simulink model "reference_block"  (R2016a)
settings: Solver=VariableStepAuto  StartTime=0.0  StopTime=10.0  RelTol=1e-3
libraries: robotlib x42
settings Model: Creator=rasrack  LastModifiedBy=rasrack

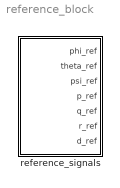
== system reference_block ==
  reference_signals : Subsystem

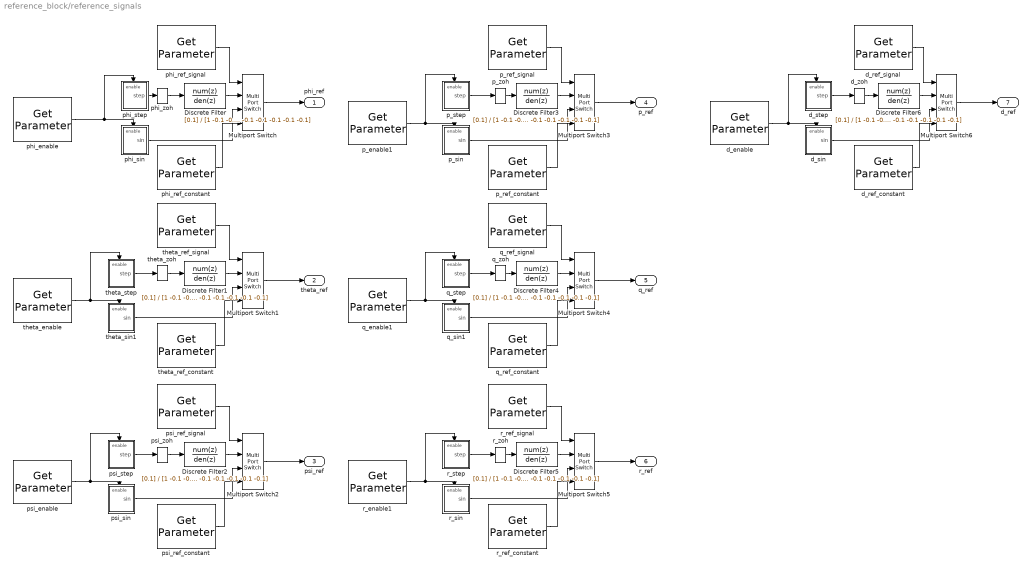
== system reference_block/reference_signals ==
  Discrete Filter{,1..6} (7 alike) : DiscreteFilter  Numerator=[0.1]  Denominator=[1 -0.1 -0.1 -0.1 -0.1 -0.1 -0.1 -0.1 -0.1 -0.1]
  Multiport Switch{,1..6} (7 alike) : MultiPortSwitch
  d_enable : robotlib/Get Parameter  SourceLibraryInfo=This block requires Robotics System Toolbox  ParameterSource=Specify your own  ParameterName=/matlab_controller/d_reference/enable  ParameterType=double  ParameterMaxArrayLength=16  ParameterInitialValue=0.0  SampleTime=-1  ShowErrorCodeOutput=off  ModelName=reference_block  BlockId=ParamGet_reference_block_242
  d_ref_constant : robotlib/Get Parameter  SourceLibraryInfo=This block requires Robotics System Toolbox  ParameterSource=Specify your own  ParameterName=/matlab_controller/d_ref_constant  ParameterType=double  ParameterMaxArrayLength=16  ParameterInitialValue=0.0  SampleTime=-1  ShowErrorCodeOutput=off  ModelName=reference_block  BlockId=ParamGet_reference_block_269
  d_ref_signal : robotlib/Get Parameter  SourceLibraryInfo=This block requires Robotics System Toolbox  ParameterSource=Specify your own  ParameterName=/matlab_controller/d_reference_signal  ParameterType=double  ParameterMaxArrayLength=16  ParameterInitialValue=0.0  SampleTime=-1  ShowErrorCodeOutput=off  ModelName=reference_block  BlockId=ParamGet_reference_block_256
  d_sin : Subsystem
  d_step : Subsystem
  d_zoh : ZeroOrderHold  SampleTime=0.010000
  p_enable1 : robotlib/Get Parameter  SourceLibraryInfo=This block requires Robotics System Toolbox  ParameterSource=Specify your own  ParameterName=/matlab_controller/p_reference/enable  ParameterType=double  ParameterMaxArrayLength=16  ParameterInitialValue=0.0  SampleTime=-1  ShowErrorCodeOutput=off  ModelName=reference_block  BlockId=ParamGet_reference_block_216
  p_ref_constant : robotlib/Get Parameter  SourceLibraryInfo=This block requires Robotics System Toolbox  ParameterSource=Specify your own  ParameterName=/matlab_controller/p_ref_constant  ParameterType=double  ParameterMaxArrayLength=16  ParameterInitialValue=0.0  SampleTime=-1  ShowErrorCodeOutput=off  ModelName=reference_block  BlockId=ParamGet_reference_block_268
  p_ref_signal : robotlib/Get Parameter  SourceLibraryInfo=This block requires Robotics System Toolbox  ParameterSource=Specify your own  ParameterName=/matlab_controller/p_reference_signal  ParameterType=double  ParameterMaxArrayLength=16  ParameterInitialValue=0.0  SampleTime=-1  ShowErrorCodeOutput=off  ModelName=reference_block  BlockId=ParamGet_reference_block_257
  p_sin : Subsystem
  p_step : Subsystem
  p_zoh : ZeroOrderHold  SampleTime=0.010000
  phi_enable : robotlib/Get Parameter  SourceLibraryInfo=This block requires Robotics System Toolbox  ParameterSource=Specify your own  ParameterName=/matlab_controller/phi_reference/enable  ParameterType=double  ParameterMaxArrayLength=16  ParameterInitialValue=0.0  SampleTime=-1  ShowErrorCodeOutput=off  ModelName=reference_block  BlockId=ParamGet_reference_block_142
  phi_ref_constant : robotlib/Get Parameter  SourceLibraryInfo=This block requires Robotics System Toolbox  ParameterSource=Specify your own  ParameterName=/matlab_controller/phi_ref_constant  ParameterType=double  ParameterMaxArrayLength=16  ParameterInitialValue=0.0  SampleTime=-1  ShowErrorCodeOutput=off  ModelName=reference_block  BlockId=ParamGet_reference_block_262
  phi_ref_signal : robotlib/Get Parameter  SourceLibraryInfo=This block requires Robotics System Toolbox  ParameterSource=Specify your own  ParameterName=/matlab_controller/phi_reference_signal  ParameterType=double  ParameterMaxArrayLength=16  ParameterInitialValue=0.0  SampleTime=-1  ShowErrorCodeOutput=off  ModelName=reference_block  BlockId=ParamGet_reference_block_255
  phi_sin : Subsystem
  phi_step : Subsystem
  phi_zoh : ZeroOrderHold  SampleTime=0.010000
  psi_enable : robotlib/Get Parameter  SourceLibraryInfo=This block requires Robotics System Toolbox  ParameterSource=Specify your own  ParameterName=/matlab_controller/psi_reference/enable  ParameterType=double  ParameterMaxArrayLength=16  ParameterInitialValue=0.0  SampleTime=-1  ShowErrorCodeOutput=off  ModelName=reference_block  BlockId=ParamGet_reference_block_164
  psi_ref_constant : robotlib/Get Parameter  SourceLibraryInfo=This block requires Robotics System Toolbox  ParameterSource=Specify your own  ParameterName=/matlab_controller/psi_ref_constant  ParameterType=double  ParameterMaxArrayLength=16  ParameterInitialValue=0.0  SampleTime=-1  ShowErrorCodeOutput=off  ModelName=reference_block  BlockId=ParamGet_reference_block_265
  psi_ref_signal : robotlib/Get Parameter  SourceLibraryInfo=This block requires Robotics System Toolbox  ParameterSource=Specify your own  ParameterName=/matlab_controller/psi_reference_signal  ParameterType=double  ParameterMaxArrayLength=16  ParameterInitialValue=0.0  SampleTime=-1  ShowErrorCodeOutput=off  ModelName=reference_block  BlockId=ParamGet_reference_block_260
  psi_sin : Subsystem
  psi_step : Subsystem
  psi_zoh : ZeroOrderHold  SampleTime=0.010000
  q_enable1 : robotlib/Get Parameter  SourceLibraryInfo=This block requires Robotics System Toolbox  ParameterSource=Specify your own  ParameterName=/matlab_controller/q_reference/enable  ParameterType=double  ParameterMaxArrayLength=16  ParameterInitialValue=0.0  SampleTime=-1  ShowErrorCodeOutput=off  ModelName=reference_block  BlockId=ParamGet_reference_block_203
  q_ref_constant : robotlib/Get Parameter  SourceLibraryInfo=This block requires Robotics System Toolbox  ParameterSource=Specify your own  ParameterName=/matlab_controller/q_ref_constant  ParameterType=double  ParameterMaxArrayLength=16  ParameterInitialValue=0.0  SampleTime=-1  ShowErrorCodeOutput=off  ModelName=reference_block  BlockId=ParamGet_reference_block_267
  q_ref_signal : robotlib/Get Parameter  SourceLibraryInfo=This block requires Robotics System Toolbox  ParameterSource=Specify your own  ParameterName=/matlab_controller/q_reference_signal  ParameterType=double  ParameterMaxArrayLength=16  ParameterInitialValue=0.0  SampleTime=-1  ShowErrorCodeOutput=off  ModelName=reference_block  BlockId=ParamGet_reference_block_258
  q_sin1 : Subsystem
  q_step : Subsystem
  q_zoh : ZeroOrderHold  SampleTime=0.010000
  r_enable1 : robotlib/Get Parameter  SourceLibraryInfo=This block requires Robotics System Toolbox  ParameterSource=Specify your own  ParameterName=/matlab_controller/r_reference/enable  ParameterType=double  ParameterMaxArrayLength=16  ParameterInitialValue=0.0  SampleTime=-1  ShowErrorCodeOutput=off  ModelName=reference_block  BlockId=ParamGet_reference_block_190
  r_ref_constant : robotlib/Get Parameter  SourceLibraryInfo=This block requires Robotics System Toolbox  ParameterSource=Specify your own  ParameterName=/matlab_controller/r_ref_constant  ParameterType=double  ParameterMaxArrayLength=16  ParameterInitialValue=0.0  SampleTime=-1  ShowErrorCodeOutput=off  ModelName=reference_block  BlockId=ParamGet_reference_block_266
  r_ref_signal : robotlib/Get Parameter  SourceLibraryInfo=This block requires Robotics System Toolbox  ParameterSource=Specify your own  ParameterName=/matlab_controller/r_reference_signal  ParameterType=double  ParameterMaxArrayLength=16  ParameterInitialValue=0.0  SampleTime=-1  ShowErrorCodeOutput=off  ModelName=reference_block  BlockId=ParamGet_reference_block_259
  r_sin : Subsystem
  r_step : Subsystem
  r_zoh : ZeroOrderHold  SampleTime=0.010000
  theta_enable : robotlib/Get Parameter  SourceLibraryInfo=This block requires Robotics System Toolbox  ParameterSource=Specify your own  ParameterName=/matlab_controller/theta_reference/enable  ParameterType=double  ParameterMaxArrayLength=16  ParameterInitialValue=0.0  SampleTime=-1  ShowErrorCodeOutput=off  ModelName=reference_block  BlockId=ParamGet_reference_block_151
  theta_ref_constant : robotlib/Get Parameter  SourceLibraryInfo=This block requires Robotics System Toolbox  ParameterSource=Specify your own  ParameterName=/matlab_controller/theta_ref_constant  ParameterType=double  ParameterMaxArrayLength=16  ParameterInitialValue=0.0  SampleTime=-1  ShowErrorCodeOutput=off  ModelName=reference_block  BlockId=ParamGet_reference_block_264
  theta_ref_signal : robotlib/Get Parameter  SourceLibraryInfo=This block requires Robotics System Toolbox  ParameterSource=Specify your own  ParameterName=/matlab_controller/theta_reference_signal  ParameterType=double  ParameterMaxArrayLength=16  ParameterInitialValue=0.0  SampleTime=-1  ShowErrorCodeOutput=off  ModelName=reference_block  BlockId=ParamGet_reference_block_261
  theta_sin1 : Subsystem
  theta_step : Subsystem
  theta_zoh : ZeroOrderHold  SampleTime=0.010000
  phi_ref : Outport
  theta_ref : Outport  Port=2
  psi_ref : Outport  Port=3
  p_ref : Outport  Port=4
  q_ref : Outport  Port=5
  r_ref : Outport  Port=6
  d_ref : Outport  Port=7
  wires:
  psi_enable/1 -> psi_step/Enable, psi_sin/Enable
  p_ref_constant/1 -> Multiport Switch3/4
  theta_ref_constant/1 -> Multiport Switch1/4
  p_sin/1(sin) -> Multiport Switch3/3
  Multiport Switch/1 -> phi_ref/1
  Discrete Filter/1 -> Multiport Switch/2
  phi_sin/1(sin) -> Multiport Switch/3
  phi_ref_signal/1 -> Multiport Switch/1
  phi_ref_constant/1 -> Multiport Switch/4
  Discrete Filter1/1 -> Multiport Switch1/2
  theta_sin1/1(sin) -> Multiport Switch1/3
  theta_ref_signal/1 -> Multiport Switch1/1
  Multiport Switch1/1 -> theta_ref/1
  Multiport Switch2/1 -> psi_ref/1
  Discrete Filter2/1 -> Multiport Switch2/2
  psi_ref_signal/1 -> Multiport Switch2/1
  Multiport Switch3/1 -> p_ref/1
  Discrete Filter3/1 -> Multiport Switch3/2
  p_ref_signal/1 -> Multiport Switch3/1
  Discrete Filter4/1 -> Multiport Switch4/2
  q_ref_signal/1 -> Multiport Switch4/1
  Multiport Switch4/1 -> q_ref/1
  Multiport Switch5/1 -> r_ref/1
  Discrete Filter5/1 -> Multiport Switch5/2
  r_ref_signal/1 -> Multiport Switch5/1
  Multiport Switch6/1 -> d_ref/1
  Discrete Filter6/1 -> Multiport Switch6/2
  d_ref_signal/1 -> Multiport Switch6/1
  phi_step/1(step) -> phi_zoh/1
  phi_zoh/1 -> Discrete Filter/1
  theta_step/1(step) -> theta_zoh/1
  theta_zoh/1 -> Discrete Filter1/1
  psi_zoh/1 -> Discrete Filter2/1
  p_zoh/1 -> Discrete Filter3/1
  q_zoh/1 -> Discrete Filter4/1
  r_zoh/1 -> Discrete Filter5/1
  d_zoh/1 -> Discrete Filter6/1
  d_sin/1(sin) -> Multiport Switch6/3
  p_enable1/1 -> p_step/Enable, p_sin/Enable
  p_step/1(step) -> p_zoh/1
  r_ref_constant/1 -> Multiport Switch5/4
  q_step/1(step) -> q_zoh/1
  phi_enable/1 -> phi_step/Enable, phi_sin/Enable
  q_ref_constant/1 -> Multiport Switch4/4
  q_sin1/1(sin) -> Multiport Switch4/3
  psi_ref_constant/1 -> Multiport Switch2/4
  d_enable/1 -> d_step/Enable, d_sin/Enable
  theta_enable/1 -> theta_step/Enable, theta_sin1/Enable
  d_step/1(step) -> d_zoh/1
  psi_sin/1(sin) -> Multiport Switch2/3
  r_enable1/1 -> r_step/Enable, r_sin/Enable
  psi_step/1(step) -> psi_zoh/1
  d_ref_constant/1 -> Multiport Switch6/4
  r_sin/1(sin) -> Multiport Switch5/3
  q_enable1/1 -> q_step/Enable, q_sin1/Enable
  r_step/1(step) -> r_zoh/1

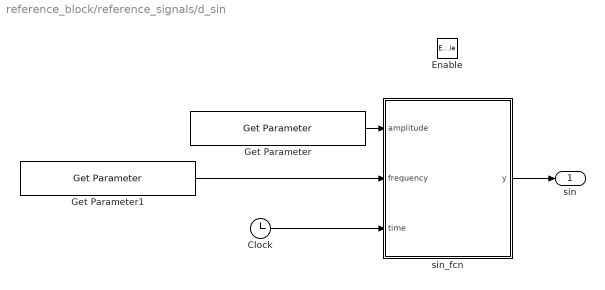
== system reference_block/reference_signals/d_sin ==
  Enable : EnablePort  StatesWhenEnabling=reset
  Clock : Clock
  Get Parameter : robotlib/Get Parameter  SourceLibraryInfo=This block requires Robotics System Toolbox  ParameterSource=Specify your own  ParameterName=/matlab_controller/d_sin/amplitude  ParameterType=double  ParameterMaxArrayLength=16  ParameterInitialValue=0.0  SampleTime=-1  ShowErrorCodeOutput=off  ModelName=reference_block  BlockId=ParamGet_reference_block_246
  Get Parameter1 : robotlib/Get Parameter  SourceLibraryInfo=This block requires Robotics System Toolbox  ParameterSource=Specify your own  ParameterName=/matlab_controller/d_sin/frequency  ParameterType=double  ParameterMaxArrayLength=16  ParameterInitialValue=0.0  SampleTime=-1  ShowErrorCodeOutput=off  ModelName=reference_block  BlockId=ParamGet_reference_block_247
  sin_fcn : MATLAB Function  TreatAsAtomicUnit=on
  sin : Outport
  wires:
  Clock/1 -> sin_fcn/3(time)
  Get Parameter1/1 -> sin_fcn/2(frequency)
  sin_fcn/1(y) -> sin/1
  Get Parameter/1 -> sin_fcn/1(amplitude)

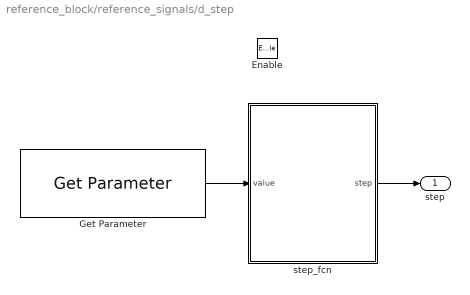
== system reference_block/reference_signals/d_step ==
  Enable : EnablePort  StatesWhenEnabling=reset
  Get Parameter : robotlib/Get Parameter  SourceLibraryInfo=This block requires Robotics System Toolbox  ParameterSource=Specify your own  ParameterName=/matlab_controller/d_step/value  ParameterType=double  ParameterMaxArrayLength=16  ParameterInitialValue=0.0  SampleTime=-1  ShowErrorCodeOutput=off  ModelName=reference_block  BlockId=ParamGet_reference_block_252
  step_fcn : MATLAB Function  TreatAsAtomicUnit=on
  step : Outport
  wires:
  step_fcn/1(step) -> step/1
  Get Parameter/1 -> step_fcn/1(value)

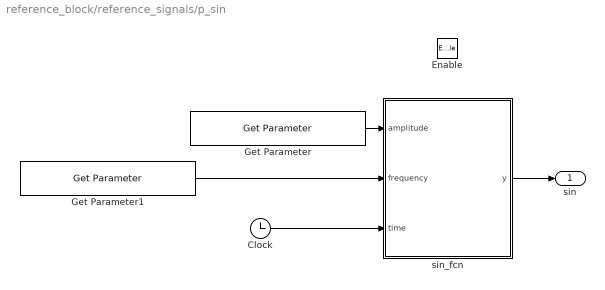
== system reference_block/reference_signals/p_sin ==
  Enable : EnablePort  StatesWhenEnabling=reset
  Clock : Clock
  Get Parameter : robotlib/Get Parameter  SourceLibraryInfo=This block requires Robotics System Toolbox  ParameterSource=Specify your own  ParameterName=/matlab_controller/p_sin/amplitude  ParameterType=double  ParameterMaxArrayLength=16  ParameterInitialValue=0.0  SampleTime=-1  ShowErrorCodeOutput=off  ModelName=reference_block  BlockId=ParamGet_reference_block_220
  Get Parameter1 : robotlib/Get Parameter  SourceLibraryInfo=This block requires Robotics System Toolbox  ParameterSource=Specify your own  ParameterName=/matlab_controller/p_sin/frequency  ParameterType=double  ParameterMaxArrayLength=16  ParameterInitialValue=0.0  SampleTime=-1  ShowErrorCodeOutput=off  ModelName=reference_block  BlockId=ParamGet_reference_block_221
  sin_fcn : MATLAB Function  TreatAsAtomicUnit=on
  sin : Outport
  wires:
  Clock/1 -> sin_fcn/3(time)
  Get Parameter1/1 -> sin_fcn/2(frequency)
  sin_fcn/1(y) -> sin/1
  Get Parameter/1 -> sin_fcn/1(amplitude)

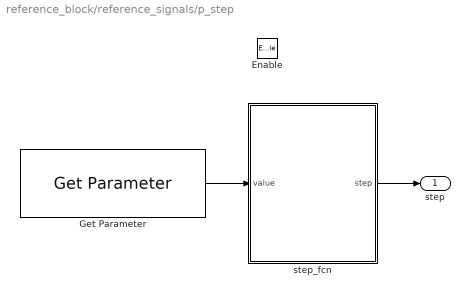
== system reference_block/reference_signals/p_step ==
  Enable : EnablePort  StatesWhenEnabling=reset
  Get Parameter : robotlib/Get Parameter  SourceLibraryInfo=This block requires Robotics System Toolbox  ParameterSource=Specify your own  ParameterName=/matlab_controller/p_step/value  ParameterType=double  ParameterMaxArrayLength=16  ParameterInitialValue=0.0  SampleTime=-1  ShowErrorCodeOutput=off  ModelName=reference_block  BlockId=ParamGet_reference_block_226
  step_fcn : MATLAB Function  TreatAsAtomicUnit=on
  step : Outport
  wires:
  step_fcn/1(step) -> step/1
  Get Parameter/1 -> step_fcn/1(value)

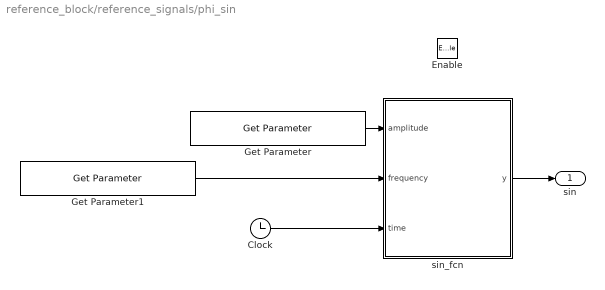
== system reference_block/reference_signals/phi_sin ==
  Enable : EnablePort  StatesWhenEnabling=reset
  Clock : Clock
  Get Parameter : robotlib/Get Parameter  SourceLibraryInfo=This block requires Robotics System Toolbox  ParameterSource=Specify your own  ParameterName=/matlab_controller/phi_sin/amplitude  ParameterType=double  ParameterMaxArrayLength=16  ParameterInitialValue=0.0  SampleTime=-1  ShowErrorCodeOutput=off  ModelName=reference_block  BlockId=ParamGet_reference_block_146
  Get Parameter1 : robotlib/Get Parameter  SourceLibraryInfo=This block requires Robotics System Toolbox  ParameterSource=Specify your own  ParameterName=/matlab_controller/phi_sin/frequency  ParameterType=double  ParameterMaxArrayLength=16  ParameterInitialValue=0.0  SampleTime=-1  ShowErrorCodeOutput=off  ModelName=reference_block  BlockId=ParamGet_reference_block_148
  sin_fcn : MATLAB Function  TreatAsAtomicUnit=on
  sin : Outport
  wires:
  Clock/1 -> sin_fcn/3(time)
  Get Parameter1/1 -> sin_fcn/2(frequency)
  sin_fcn/1(y) -> sin/1
  Get Parameter/1 -> sin_fcn/1(amplitude)

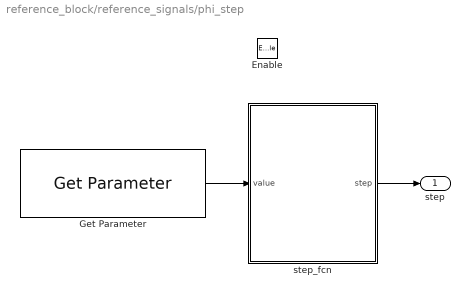
== system reference_block/reference_signals/phi_step ==
  Enable : EnablePort  StatesWhenEnabling=reset
  Get Parameter : robotlib/Get Parameter  SourceLibraryInfo=This block requires Robotics System Toolbox  ParameterSource=Specify your own  ParameterName=/matlab_controller/phi_step/value  ParameterType=double  ParameterMaxArrayLength=16  ParameterInitialValue=0.0  SampleTime=-1  ShowErrorCodeOutput=off  ModelName=reference_block  BlockId=ParamGet_reference_block_141
  step_fcn : MATLAB Function  TreatAsAtomicUnit=on
  step : Outport
  wires:
  step_fcn/1(step) -> step/1
  Get Parameter/1 -> step_fcn/1(value)

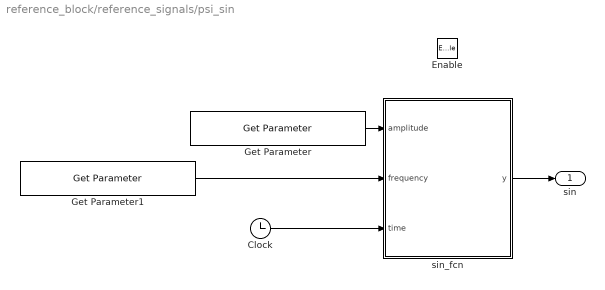
== system reference_block/reference_signals/psi_sin ==
  Enable : EnablePort  StatesWhenEnabling=reset
  Clock : Clock
  Get Parameter : robotlib/Get Parameter  SourceLibraryInfo=This block requires Robotics System Toolbox  ParameterSource=Specify your own  ParameterName=/matlab_controller/psi_sin/amplitude  ParameterType=double  ParameterMaxArrayLength=16  ParameterInitialValue=0.0  SampleTime=-1  ShowErrorCodeOutput=off  ModelName=reference_block  BlockId=ParamGet_reference_block_168
  Get Parameter1 : robotlib/Get Parameter  SourceLibraryInfo=This block requires Robotics System Toolbox  ParameterSource=Specify your own  ParameterName=/matlab_controller/psi_sin/frequency  ParameterType=double  ParameterMaxArrayLength=16  ParameterInitialValue=0.0  SampleTime=-1  ShowErrorCodeOutput=off  ModelName=reference_block  BlockId=ParamGet_reference_block_169
  sin_fcn : MATLAB Function  TreatAsAtomicUnit=on
  sin : Outport
  wires:
  Clock/1 -> sin_fcn/3(time)
  Get Parameter1/1 -> sin_fcn/2(frequency)
  sin_fcn/1(y) -> sin/1
  Get Parameter/1 -> sin_fcn/1(amplitude)

== system reference_block/reference_signals/psi_step ==
  Enable : EnablePort  StatesWhenEnabling=reset
  Get Parameter : robotlib/Get Parameter  SourceLibraryInfo=This block requires Robotics System Toolbox  ParameterSource=Specify your own  ParameterName=/matlab_controller/psi_step/value  ParameterType=double  ParameterMaxArrayLength=16  ParameterInitialValue=0.0  SampleTime=-1  ShowErrorCodeOutput=off  ModelName=reference_block  BlockId=ParamGet_reference_block_174
  step_fcn : MATLAB Function  TreatAsAtomicUnit=on
  step : Outport
  wires:
  step_fcn/1(step) -> step/1
  Get Parameter/1 -> step_fcn/1(value)

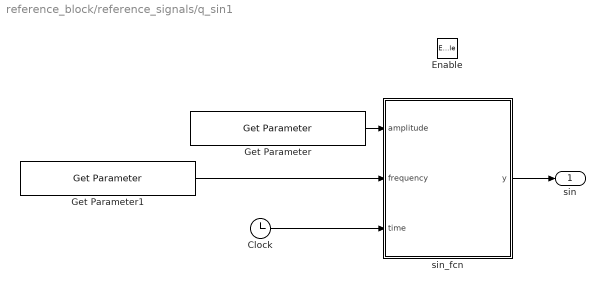
== system reference_block/reference_signals/q_sin1 ==
  Enable : EnablePort  StatesWhenEnabling=reset
  Clock : Clock
  Get Parameter : robotlib/Get Parameter  SourceLibraryInfo=This block requires Robotics System Toolbox  ParameterSource=Specify your own  ParameterName=/matlab_controller/q_sin/amplitude  ParameterType=double  ParameterMaxArrayLength=16  ParameterInitialValue=0.0  SampleTime=-1  ShowErrorCodeOutput=off  ModelName=reference_block  BlockId=ParamGet_reference_block_207
  Get Parameter1 : robotlib/Get Parameter  SourceLibraryInfo=This block requires Robotics System Toolbox  ParameterSource=Specify your own  ParameterName=/matlab_controller/q_sin/frequency  ParameterType=double  ParameterMaxArrayLength=16  ParameterInitialValue=0.0  SampleTime=-1  ShowErrorCodeOutput=off  ModelName=reference_block  BlockId=ParamGet_reference_block_208
  sin_fcn : MATLAB Function  TreatAsAtomicUnit=on
  sin : Outport
  wires:
  Clock/1 -> sin_fcn/3(time)
  Get Parameter1/1 -> sin_fcn/2(frequency)
  sin_fcn/1(y) -> sin/1
  Get Parameter/1 -> sin_fcn/1(amplitude)

== system reference_block/reference_signals/q_step ==
  Enable : EnablePort  StatesWhenEnabling=reset
  Get Parameter : robotlib/Get Parameter  SourceLibraryInfo=This block requires Robotics System Toolbox  ParameterSource=Specify your own  ParameterName=/matlab_controller/q_step/value  ParameterType=double  ParameterMaxArrayLength=16  ParameterInitialValue=0.0  SampleTime=-1  ShowErrorCodeOutput=off  ModelName=reference_block  BlockId=ParamGet_reference_block_213
  step_fcn : MATLAB Function  TreatAsAtomicUnit=on
  step : Outport
  wires:
  step_fcn/1(step) -> step/1
  Get Parameter/1 -> step_fcn/1(value)

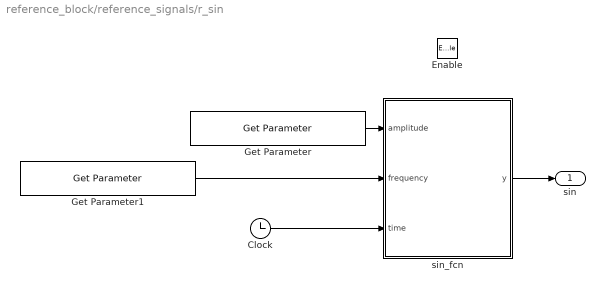
== system reference_block/reference_signals/r_sin ==
  Enable : EnablePort  StatesWhenEnabling=reset
  Clock : Clock
  Get Parameter : robotlib/Get Parameter  SourceLibraryInfo=This block requires Robotics System Toolbox  ParameterSource=Specify your own  ParameterName=/matlab_controller/r_sin/amplitude  ParameterType=double  ParameterMaxArrayLength=16  ParameterInitialValue=0.0  SampleTime=-1  ShowErrorCodeOutput=off  ModelName=reference_block  BlockId=ParamGet_reference_block_194
  Get Parameter1 : robotlib/Get Parameter  SourceLibraryInfo=This block requires Robotics System Toolbox  ParameterSource=Specify your own  ParameterName=/matlab_controller/r_sin/frequency  ParameterType=double  ParameterMaxArrayLength=16  ParameterInitialValue=0.0  SampleTime=-1  ShowErrorCodeOutput=off  ModelName=reference_block  BlockId=ParamGet_reference_block_195
  sin_fcn : MATLAB Function  TreatAsAtomicUnit=on
  sin : Outport
  wires:
  Clock/1 -> sin_fcn/3(time)
  Get Parameter1/1 -> sin_fcn/2(frequency)
  sin_fcn/1(y) -> sin/1
  Get Parameter/1 -> sin_fcn/1(amplitude)

== system reference_block/reference_signals/r_step ==
  Enable : EnablePort  StatesWhenEnabling=reset
  Get Parameter : robotlib/Get Parameter  SourceLibraryInfo=This block requires Robotics System Toolbox  ParameterSource=Specify your own  ParameterName=/matlab_controller/r_step/value  ParameterType=double  ParameterMaxArrayLength=16  ParameterInitialValue=0.0  SampleTime=-1  ShowErrorCodeOutput=off  ModelName=reference_block  BlockId=ParamGet_reference_block_200
  step_fcn : MATLAB Function  TreatAsAtomicUnit=on
  step : Outport
  wires:
  step_fcn/1(step) -> step/1
  Get Parameter/1 -> step_fcn/1(value)

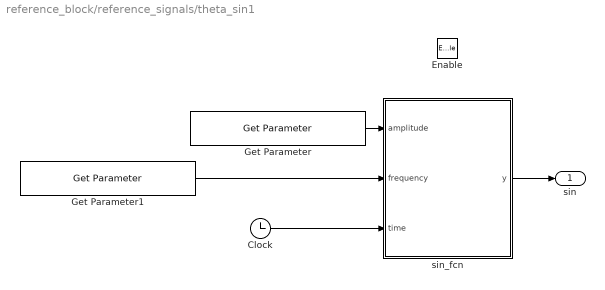
== system reference_block/reference_signals/theta_sin1 ==
  Enable : EnablePort  StatesWhenEnabling=reset
  Clock : Clock
  Get Parameter : robotlib/Get Parameter  SourceLibraryInfo=This block requires Robotics System Toolbox  ParameterSource=Specify your own  ParameterName=/matlab_controller/theta_sin/amplitude  ParameterType=double  ParameterMaxArrayLength=16  ParameterInitialValue=0.0  SampleTime=-1  ShowErrorCodeOutput=off  ModelName=reference_block  BlockId=ParamGet_reference_block_155
  Get Parameter1 : robotlib/Get Parameter  SourceLibraryInfo=This block requires Robotics System Toolbox  ParameterSource=Specify your own  ParameterName=/matlab_controller/theta_sin/frequency  ParameterType=double  ParameterMaxArrayLength=16  ParameterInitialValue=0.0  SampleTime=-1  ShowErrorCodeOutput=off  ModelName=reference_block  BlockId=ParamGet_reference_block_156
  sin_fcn : MATLAB Function  TreatAsAtomicUnit=on
  sin : Outport
  wires:
  Clock/1 -> sin_fcn/3(time)
  Get Parameter1/1 -> sin_fcn/2(frequency)
  sin_fcn/1(y) -> sin/1
  Get Parameter/1 -> sin_fcn/1(amplitude)

== system reference_block/reference_signals/theta_step ==
  Enable : EnablePort  StatesWhenEnabling=reset
  Get Parameter : robotlib/Get Parameter  SourceLibraryInfo=This block requires Robotics System Toolbox  ParameterSource=Specify your own  ParameterName=/matlab_controller/theta_step/value  ParameterType=double  ParameterMaxArrayLength=16  ParameterInitialValue=0.0  SampleTime=-1  ShowErrorCodeOutput=off  ModelName=reference_block  BlockId=ParamGet_reference_block_161
  step_fcn : MATLAB Function  TreatAsAtomicUnit=on
  step : Outport
  wires:
  step_fcn/1(step) -> step/1
  Get Parameter/1 -> step_fcn/1(value)

== matlab function reference_block/reference_signals/theta_sin1/sin_fcn ==
  data: amplitude input; y output; frequency input; time input
function y = fcn(amplitude, frequency, time)
%#codegen

y = amplitude*sin(frequency*time);

end

== matlab function reference_block/reference_signals/theta_step/step_fcn ==
  data: step output; value input
function step = fcn(value)
%#codegen


step = value;

end

== matlab function reference_block/reference_signals/psi_sin/sin_fcn ==
  data: amplitude input; y output; frequency input; time input
function y = fcn(amplitude, frequency, time)
%#codegen

y = amplitude*sin(frequency*time);

end

== matlab function reference_block/reference_signals/psi_step/step_fcn ==
  data: step output; value input
function step = fcn(value)
%#codegen


step = value;

end

== matlab function reference_block/reference_signals/r_sin/sin_fcn ==
  data: amplitude input; y output; frequency input; time input
function y = fcn(amplitude, frequency, time)
%#codegen

y = amplitude*sin(frequency*time);

end

== matlab function reference_block/reference_signals/r_step/step_fcn ==
  data: step output; value input
function step = fcn(value)
%#codegen


step = value;

end

== matlab function reference_block/reference_signals/q_sin1/sin_fcn ==
  data: amplitude input; y output; frequency input; time input
function y = fcn(amplitude, frequency, time)
%#codegen

y = amplitude*sin(frequency*time);

end

== matlab function reference_block/reference_signals/q_step/step_fcn ==
  data: step output; value input
function step = fcn(value)
%#codegen


step = value;

end

== matlab function reference_block/reference_signals/p_sin/sin_fcn ==
  data: amplitude input; y output; frequency input; time input
function y = fcn(amplitude, frequency, time)
%#codegen

y = amplitude*sin(frequency*time);

end

== matlab function reference_block/reference_signals/p_step/step_fcn ==
  data: step output; value input
function step = fcn(value)
%#codegen


step = value;

end

== matlab function reference_block/reference_signals/d_sin/sin_fcn ==
  data: amplitude input; y output; frequency input; time input
function y = fcn(amplitude, frequency, time)
%#codegen

y = amplitude*sin(frequency*time);

end

== matlab function reference_block/reference_signals/d_step/step_fcn ==
  data: step output; value input
function step = fcn(value)
%#codegen


step = value;

end

== matlab function reference_block/reference_signals/phi_step/step_fcn ==
  data: step output; value input
function step = fcn(value)
%#codegen


step = value;

end

== matlab function reference_block/reference_signals/phi_sin/sin_fcn ==
  data: amplitude input; y output; frequency input; time input
function y = fcn(amplitude, frequency, time)
%#codegen

y = amplitude*sin(frequency*time);

end
